simulink model "rul_data_acquisition_complete_needs_debugging"  (R2023b)
settings: Solver=FixedStepAuto  StartTime=0.0  StopTime=Inf  RelTol=1e-3  EnableMultiTasking=on
model workspace (MAT data in the model file):
  rul_data = [1 1]
libraries: c2802xlib x4
settings Model: ExtModeTrigDuration=8  Creator=Yamukelani  LastModifiedBy=yamzi
settings DataIOCC: InspectSignalLogs=on  LoggingToFile=on  LoggingFileName=rul_data.csv
settings OptimizationCC: DefaultUnderspecifiedDataType=single  EnhancedBackFolding=on  PassReuseOutputArgsAs=Individual arguments  MaxStackSize=768  OptimizeBlockOrder=speed  DifferentSizesBufferReuse=on  OptimizationCustomize=off  EfficientTunableParamExpr=on
settings DebuggingCC: ParameterTunabilityLossMsg=error
settings HardwareCC: ProdBitPerChar=16  ProdBitPerInt=16  ProdBitPerPointer=32  ProdBitPerSizeT=32  ProdBitPerPtrDiffT=32  ProdLargestAtomicInteger=Integer  ProdLargestAtomicFloat=None  ProdWordSize=16  ProdLongLongMode=on  ProdHWDeviceType=Texas Instruments->C2000
settings ModelReferenceCC: ModelReferenceNumInstancesAllowed=Single
settings SFSimCC: MATLABDynamicMemAlloc=off
settings RTWCC: Description=Embedded Coder  SystemTargetFile=ert.tlc  HardwareBoard=TI Piccolo F28027/F28027F LaunchPad  TemplateMakefile=ert_default_tmf  Toolchain=Texas Instruments Code Composer Studio (C2000)  CodeProfilingSaveOptions=MetricsOnly
settings CodeAppCC: ForceParamTrailComments=on  IgnoreCustomStorageClasses=off  OperatorAnnotations=on  SimulinkDataObjDesc=on  SFDataObjDesc=on  InsertBlockDesc=on
settings ERTTargetCC: CodeReplacementLibrary=TI C28x  ExtModeTransport=4  ExtModeStaticAlloc=on  ExtModeAutomaticAllocSize=off  ExtModeStaticAllocSize=500  ExtModeMexFile=ext_xcp  ExtModeIntrfLevel=Level2 - Open

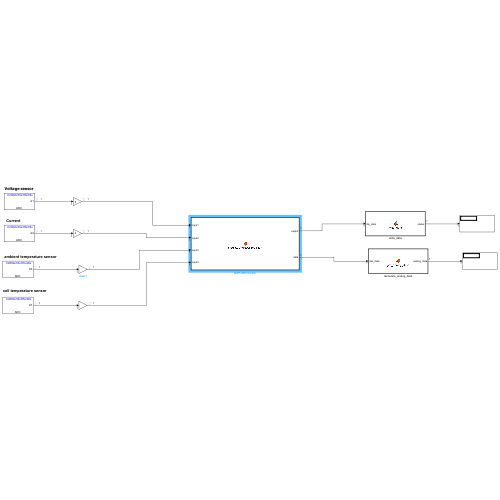
[thumbnail: Simulink's stored preview of the top-level diagram]
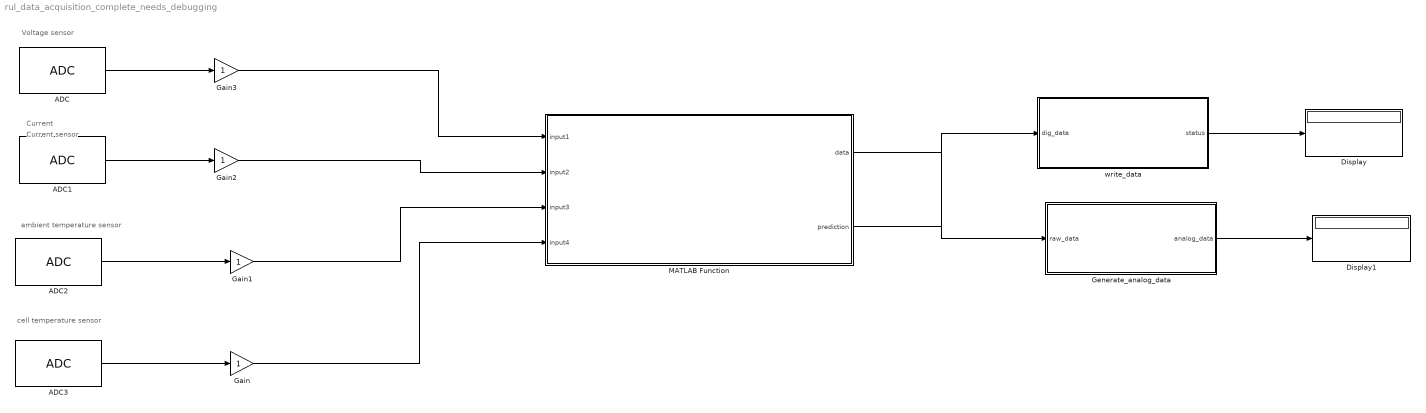
== system rul_data_acquisition_complete_needs_debugging ==
  note: Current
  note: Current sensor
  note: Voltage sensor
  note: ambient temperature sensor
  note: cell temperature sensor
  ADC : c2802xlib/ADC  blkParamProc=C2000  ADCModule=1  samplingMode=Single sample mode  ADCResolution=12-bit (Single-ended input)  useSOC1=SOC0  useSOC2=SOC0_SOC1  SOCAcquisitionWindow=7  SOCTriggerSource=CPU0_TINT0n  SOCInterruptTrigger=ADCINT1  Ts=0.005  dType=int16  postInterrupt=off  interruptSel=ADCINT1  ADCINTContinuous=on  endma=off  chdma=1  conv1=ADCINA1  conv2=ADCINA0 and ADCINB0  conv1_Type4=ADCIN0  conv2_Type4=ADCIN0 and ADCIN1
  ADC1 : c2802xlib/ADC  blkParamProc=C2000  ADCModule=1  samplingMode=Single sample mode  ADCResolution=12-bit (Single-ended input)  useSOC1=SOC1  useSOC2=SOC0_SOC1  SOCAcquisitionWindow=7  SOCTriggerSource=CPU1_TINT1n  SOCInterruptTrigger=ADCINT1  Ts=0.005  dType=uint16  postInterrupt=off  interruptSel=ADCINT1  ADCINTContinuous=on  endma=off  chdma=1  conv1=ADCINA2  conv2=ADCINA0 and ADCINB0  conv1_Type4=ADCIN0  conv2_Type4=ADCIN0 and ADCIN1
  ADC2 : c2802xlib/ADC  blkParamProc=C2000  ADCModule=1  samplingMode=Single sample mode  ADCResolution=12-bit (Single-ended input)  useSOC1=SOC2  useSOC2=SOC0_SOC1  SOCAcquisitionWindow=7  SOCTriggerSource=CPU2_TINT2n  SOCInterruptTrigger=ADCINT2  Ts=0.005  dType=uint16  postInterrupt=off  interruptSel=ADCINT1  ADCINTContinuous=on  endma=off  chdma=1  conv1=ADCINA3  conv2=ADCINA0 and ADCINB0  conv1_Type4=ADCIN0  conv2_Type4=ADCIN0 and ADCIN1
  ADC3 : c2802xlib/ADC  blkParamProc=C2000  ADCModule=1  samplingMode=Single sample mode  ADCResolution=12-bit (Single-ended input)  useSOC1=SOC3  useSOC2=SOC0_SOC1  SOCAcquisitionWindow=7  SOCTriggerSource=ePWM1_ADCSOCA  SOCInterruptTrigger=No ADCINT  Ts=0.005  dType=int16  postInterrupt=off  interruptSel=ADCINT1  ADCINTContinuous=on  endma=off  chdma=1  conv1=ADCINA7  conv2=ADCINA0 and ADCINB0  conv1_Type4=ADCIN0  conv2_Type4=ADCIN0 and ADCIN1
  Display : Display
  Display1 : Display
  Gain{,1..3} (4 alike) : Gain
  Generate_analog_data : MATLAB Function  TreatAsAtomicUnit=on
  MATLAB Function : MATLAB Function  TreatAsAtomicUnit=on
  write_data : MATLAB Function  TreatAsAtomicUnit=on
  wires:
  ADC3/1 -> Gain/1
  ADC2/1 -> Gain1/1
  ADC1/1 -> Gain2/1
  ADC/1 -> Gain3/1
  Gain3/1 -> MATLAB Function/1(input1)
  Gain2/1 -> MATLAB Function/2(input2)
  Gain1/1 -> MATLAB Function/3(input3)
  Gain/1 -> MATLAB Function/4(input4)
  MATLAB Function/2(prediction) -> write_data/1(dig_data)
  MATLAB Function/1(data) -> Generate_analog_data/1(raw_data)
  write_data/1(status) -> Display/1
  Generate_analog_data/1(analog_data) -> Display1/1

== matlab function rul_data_acquisition_complete_needs_debugging/write_data ==
  data: dig_data input; status output
function status = write_data(dig_data)
%Wite data to a file
writecell( dig_data, 'C:\Users\yamzi\OneDrive\Documents\Master in Science Research\Battery life prediction\data\sensor_data.csv');
status = 0;

== matlab function rul_data_acquisition_complete_needs_debugging/Generate_analog_data ==
  data: raw_data input; analog_data output
function analog_data = get_analog_data(raw_data)
%Get the required paramters.
raw_voltage = raw_data(0);
raw_current = raw_data(1);
cell_temperature = raw_data(2);
amb_temperature = raw_data(3);

%Calculate analog voltage
resistor1 = 30000.0; 
resistor2 = 7500.0;
vout = (raw_voltage * 5.0) / 1024.0; % see datasheet
voltage = vout / (resistor2/(resistor1+resistor2));

%Calculate analog current
mv_per_amp = 66;
current_val = (raw_current / 1024.0) * 5000; % Calculates the mV
acs_offset = 2500; 
current = ((current_val - acs_offset) / mv_per_amp);

analog_data = [voltage, current,cell_temperature, amb_temperature];

== matlab function rul_data_acquisition_complete_needs_debugging/MATLAB Function ==
  data: data output; input1 input; prediction output; input2 input; input3 input; input4 input
function [data,prediction]= predictUsingRULPrediction(input1, input2, input3, input4)
    % Load the pre-trained TreeBagger model
    coder.extrinsic("predict")
    data = [input1,input2,input3,input4];
    rul_pred_model = load("C:\Users\yamzi\source_code\msc_research\rul_prediction\src\matlab_code\models\gpr_rul_model.mat"', 'RULPredModel');
    % Make predictions using the loaded model
    prediction = predict(rul_pred_model, data);
end
